simulink model "ackerman_ROS_neural_controller_v2"  (R2023a)
settings: Solver=FixedStepDiscrete  StartTime=0.0  StopTime=200  FixedStep=0.1  RelTol=1e-3
undefined symbols (not defined in the file or in its folder): Angular, Linear
libraries: neural x413, robotlib x15, robotcorelib x1
(part 8 of 17)

== system ackerman_ROS_neural_controller_v2/ME ENCANTA/Layer 1/IW{1,1} ==
  "pd{1,1}" : Inport  PortDimensions=8  SampleTime=0.1
      mask Display: e = 0.06;c1 = [120 230 180]/255;c2 = ([120 230 180]+0)/(256+128);c3 = ([120 230 180]+128)/(256+128);patch([0 1 1 0],[0 0 1 1],c1);patch([0 1 1 1-e 1-e 0+e],[0 0 1 1-e 0+e 0+e],c2);patch([0 0 1 1-e 0+e 0+e],[0 1 1 1-e 1-e 0+e],c3);plot([0 1 1 0 0],[0 0 1 1 0]);
  "IW{1,1}(1,:)'" : Constant  Value=[0.971980235182158924800432941992767155170440673828125;2.567078221588861453028584946878254413604736328125;-0.0638964923073234991601765386803890578448772430419921875;0.187982900118411178080890522323898039758205413818359375;1.435142271716796091851620076340623199939727783203125;-1.2440064926958480651109084647032432258129119873046875;-1.715625221300081104658374897553585469722747802734375;-0.3178705401241617156671281918534077703952789306640625]
      mask Display: e = 0.06;c1 = [120 150 230]/255;c2 = ([120 150 230]+0)/383;c3 = ([120 150 230]+128)/383;patch([0 1 1 0],[0 0 1 1],c1);patch([0 1 1 1-e 1-e 0+e],[0 0 1 1-e 0+e 0+e],c2);patch([0 0 1 1-e 0+e 0+e],[0 1 1 1-e 1-e 0+e],c3);plot([0 1 1 0 0],[0 0 1 1 0]);disp('Weights');
  "IW{1,1}(10,:)'" : Constant  Value=[0.952957574863269929466014218633063137531280517578125;-1.279752017667800334521643890184350311756134033203125;-0.780817996752551923833607361302711069583892822265625;-0.73631471257776326400090738388826139271259307861328125;0.279679452980061415967583116071182303130626678466796875;1.76479096051938189049224092741496860980987548828125;-0.41872113667667931746763088085572235286235809326171875;-0.269270961130175290332289250727626495063304901123046875]
      mask Display: e = 0.06;c1 = [120 150 230]/255;c2 = ([120 150 230]+0)/383;c3 = ([120 150 230]+128)/383;patch([0 1 1 0],[0 0 1 1],c1);patch([0 1 1 1-e 1-e 0+e],[0 0 1 1-e 0+e 0+e],c2);patch([0 0 1 1-e 0+e 0+e],[0 1 1 1-e 1-e 0+e],c3);plot([0 1 1 0 0],[0 0 1 1 0]);disp('Weights');
  "IW{1,1}(11,:)'" : Constant  Value=[-0.7943142555522564318692957385792396962642669677734375;-0.54810133824739093455491456552408635616302490234375;-0.0209028643619187902424894076602868153713643550872802734375;0.207116084413179468715071607221034355461597442626953125;1.4609012214747443270113080870942212641239166259765625;-0.94419545667940074640256398197379894554615020751953125;-1.49407969221122893799247322021983563899993896484375;0.36046049644091560093528414654429070651531219482421875]
      mask Display: e = 0.06;c1 = [120 150 230]/255;c2 = ([120 150 230]+0)/383;c3 = ([120 150 230]+128)/383;patch([0 1 1 0],[0 0 1 1],c1);patch([0 1 1 1-e 1-e 0+e],[0 0 1 1-e 0+e 0+e],c2);patch([0 0 1 1-e 0+e 0+e],[0 1 1 1-e 1-e 0+e],c3);plot([0 1 1 0 0],[0 0 1 1 0]);disp('Weights');
  "IW{1,1}(12,:)'" : Constant  Value=[-1.63964337746614763346997278858907520771026611328125;0.60076169030219350730703808949328958988189697265625;0.71625941833236861366884795643272809684276580810546875;0.28432619515038293211972586504998616874217987060546875;1.008858171661137337338232100591994822025299072265625;1.226017776539758852294426105800084769725799560546875;-1.7365630219620447061146251144236885011196136474609375;-0.429447135602839313861522896331734955310821533203125]
      mask Display: e = 0.06;c1 = [120 150 230]/255;c2 = ([120 150 230]+0)/383;c3 = ([120 150 230]+128)/383;patch([0 1 1 0],[0 0 1 1],c1);patch([0 1 1 1-e 1-e 0+e],[0 0 1 1-e 0+e 0+e],c2);patch([0 0 1 1-e 0+e 0+e],[0 1 1 1-e 1-e 0+e],c3);plot([0 1 1 0 0],[0 0 1 1 0]);disp('Weights');
  "IW{1,1}(13,:)'" : Constant  Value=[-0.046458660075713177628475847313893609680235385894775390625;1.309328092935980958344543978455476462841033935546875;-0.2053412555322882138142404073732905089855194091796875;-1.0241502298471925058720444212667644023895263671875;0.33819473753734718979302442676271311938762664794921875;1.500511362857012809257639673887751996517181396484375;0.89838152047738495387108059730962850153446197509765625;0.38963898857398138186880487410235218703746795654296875]
      mask Display: e = 0.06;c1 = [120 150 230]/255;c2 = ([120 150 230]+0)/383;c3 = ([120 150 230]+128)/383;patch([0 1 1 0],[0 0 1 1],c1);patch([0 1 1 1-e 1-e 0+e],[0 0 1 1-e 0+e 0+e],c2);patch([0 0 1 1-e 0+e 0+e],[0 1 1 1-e 1-e 0+e],c3);plot([0 1 1 0 0],[0 0 1 1 0]);disp('Weights');
  "IW{1,1}(14,:)'" : Constant  Value=[-0.835126481572200152214691115659661591053009033203125;0.67771081724395265677429733841563574969768524169921875;0.32746319190107009422519013241981156170368194580078125;0.496135681159649621907448135971208103001117706298828125;-0.77500849546231187492395520166610367596149444580078125;-0.53766641721378238827355744433589279651641845703125;0.354972473239116237397894337846082635223865509033203125;1.312743418109337145693871207186020910739898681640625]
      mask Display: e = 0.06;c1 = [120 150 230]/255;c2 = ([120 150 230]+0)/383;c3 = ([120 150 230]+128)/383;patch([0 1 1 0],[0 0 1 1],c1);patch([0 1 1 1-e 1-e 0+e],[0 0 1 1-e 0+e 0+e],c2);patch([0 0 1 1-e 0+e 0+e],[0 1 1 1-e 1-e 0+e],c3);plot([0 1 1 0 0],[0 0 1 1 0]);disp('Weights');
  "IW{1,1}(15,:)'" : Constant  Value=[-0.18608216993497517233180360562982968986034393310546875;-0.67339069859827649366934565478004515171051025390625;0.286183692221986085701956881166552193462848663330078125;0.90019583556312310346214644596329890191555023193359375;-1.424886791004641661828600263106636703014373779296875;-0.552278192782113652725684005417861044406890869140625;-0.58322513421994226501254843242350034415721893310546875;0.71811307953740766141237372721661813557147979736328125]
      mask Display: e = 0.06;c1 = [120 150 230]/255;c2 = ([120 150 230]+0)/383;c3 = ([120 150 230]+128)/383;patch([0 1 1 0],[0 0 1 1],c1);patch([0 1 1 1-e 1-e 0+e],[0 0 1 1-e 0+e 0+e],c2);patch([0 0 1 1-e 0+e 0+e],[0 1 1 1-e 1-e 0+e],c3);plot([0 1 1 0 0],[0 0 1 1 0]);disp('Weights');
  "IW{1,1}(2,:)'" : Constant  Value=[-1.35611856667662333819635023246519267559051513671875;-0.6596259355066333984751736352336592972278594970703125;-2.15308333009377150801810785196721553802490234375;-0.594254710313253386999576832749880850315093994140625;1.183809903206018088184237058158032596111297607421875;1.3778074261582233805967234729905612766742706298828125;-0.4951736029469759881038726234692148864269256591796875;-0.5083250892003707832600412075407803058624267578125]
      mask Display: e = 0.06;c1 = [120 150 230]/255;c2 = ([120 150 230]+0)/383;c3 = ([120 150 230]+128)/383;patch([0 1 1 0],[0 0 1 1],c1);patch([0 1 1 1-e 1-e 0+e],[0 0 1 1-e 0+e 0+e],c2);patch([0 0 1 1-e 0+e 0+e],[0 1 1 1-e 1-e 0+e],c3);plot([0 1 1 0 0],[0 0 1 1 0]);disp('Weights');
  "IW{1,1}(3,:)'" : Constant  Value=[0.389330121892868863398007306386716663837432861328125;0.2289315734305190641606486678938381373882293701171875;0.68045717842820419019034261509659700095653533935546875;-0.72428464448281071330626446069800294935703277587890625;-3.111683839695417841397784286527894437313079833984375;1.8061369740664001692920237474027089774608612060546875;2.901306769919713257621651791851036250591278076171875;-0.165240155407275712828862879177904687821865081787109375]
      mask Display: e = 0.06;c1 = [120 150 230]/255;c2 = ([120 150 230]+0)/383;c3 = ([120 150 230]+128)/383;patch([0 1 1 0],[0 0 1 1],c1);patch([0 1 1 1-e 1-e 0+e],[0 0 1 1-e 0+e 0+e],c2);patch([0 0 1 1-e 0+e 0+e],[0 1 1 1-e 1-e 0+e],c3);plot([0 1 1 0 0],[0 0 1 1 0]);disp('Weights');
  "IW{1,1}(4,:)'" : Constant  Value=[1.6848774452106629606618071193224750459194183349609375;-0.2113971201403252175854419192546629346907138824462890625;-0.40644343158014095696017875525285489857196807861328125;0.98312175830758985473067923521739430725574493408203125;1.5222720525634070298792721587233245372772216796875;0.37693409531385524413593657300225459039211273193359375;0.2450165084343079169304502329396200366318225860595703125;-0.760503980708643556596371126943267881870269775390625]
      mask Display: e = 0.06;c1 = [120 150 230]/255;c2 = ([120 150 230]+0)/383;c3 = ([120 150 230]+128)/383;patch([0 1 1 0],[0 0 1 1],c1);patch([0 1 1 1-e 1-e 0+e],[0 0 1 1-e 0+e 0+e],c2);patch([0 0 1 1-e 0+e 0+e],[0 1 1 1-e 1-e 0+e],c3);plot([0 1 1 0 0],[0 0 1 1 0]);disp('Weights');
  "IW{1,1}(5,:)'" : Constant  Value=[1.7316373522789654249010027342592366039752960205078125;1.2495315454890889572681089703110046684741973876953125;1.1345171396436393163043021559133194386959075927734375;0.55816746854987309145457174963667057454586029052734375;0.336413043621611784761427088596974499523639678955078125;-0.6475244665177035674474836923764087259769439697265625;1.2412636084071022590791244510910473763942718505859375;-0.45205615342753124874519699005759321153163909912109375]
      mask Display: e = 0.06;c1 = [120 150 230]/255;c2 = ([120 150 230]+0)/383;c3 = ([120 150 230]+128)/383;patch([0 1 1 0],[0 0 1 1],c1);patch([0 1 1 1-e 1-e 0+e],[0 0 1 1-e 0+e 0+e],c2);patch([0 0 1 1-e 0+e 0+e],[0 1 1 1-e 1-e 0+e],c3);plot([0 1 1 0 0],[0 0 1 1 0]);disp('Weights');
  "IW{1,1}(6,:)'" : Constant  Value=[-0.1509239964485774854185962112751440145075321197509765625;-1.19586695150943089771544691757299005985260009765625;0.80360230515575514775861165617243386805057525634765625;-0.6183180438151278934810761711560189723968505859375;1.2181859235617549241936785620055161416530609130859375;-1.402058986093745573953128769062459468841552734375;2.21178431671591813056920727831311523914337158203125;5.8493224896000324264377923100255429744720458984375]
      mask Display: e = 0.06;c1 = [120 150 230]/255;c2 = ([120 150 230]+0)/383;c3 = ([120 150 230]+128)/383;patch([0 1 1 0],[0 0 1 1],c1);patch([0 1 1 1-e 1-e 0+e],[0 0 1 1-e 0+e 0+e],c2);patch([0 0 1 1-e 0+e 0+e],[0 1 1 1-e 1-e 0+e],c3);plot([0 1 1 0 0],[0 0 1 1 0]);disp('Weights');
  "IW{1,1}(7,:)'" : Constant  Value=[0.8609195814912504740590293295099399983882904052734375;-2.130317054986762048685022818972356617450714111328125;-0.056947587820770355360178172077212366275489330291748046875;0.327433012969035319716937237899401225149631500244140625;0.2186081327389498285551638900869875214993953704833984375;-1.036658261972080996571321520605124533176422119140625;2.47996978858621286434527064557187259197235107421875;-1.953257557304577840540105171385221183300018310546875]
      mask Display: e = 0.06;c1 = [120 150 230]/255;c2 = ([120 150 230]+0)/383;c3 = ([120 150 230]+128)/383;patch([0 1 1 0],[0 0 1 1],c1);patch([0 1 1 1-e 1-e 0+e],[0 0 1 1-e 0+e 0+e],c2);patch([0 0 1 1-e 0+e 0+e],[0 1 1 1-e 1-e 0+e],c3);plot([0 1 1 0 0],[0 0 1 1 0]);disp('Weights');
  "IW{1,1}(8,:)'" : Constant  Value=[-0.46388264526166789192274109154823236167430877685546875;-0.5661191272907097893352101891650818288326263427734375;-0.181870215050510652954329771091579459607601165771484375;0.300246660440473822628604239071137271821498870849609375;-0.025378748936564408944516202382146730087697505950927734375;1.61731333714226455100515522644855082035064697265625;1.5124425407989434688715846277773380279541015625;-0.1772881404680668737672277757155825383961200714111328125]
      mask Display: e = 0.06;c1 = [120 150 230]/255;c2 = ([120 150 230]+0)/383;c3 = ([120 150 230]+128)/383;patch([0 1 1 0],[0 0 1 1],c1);patch([0 1 1 1-e 1-e 0+e],[0 0 1 1-e 0+e 0+e],c2);patch([0 0 1 1-e 0+e 0+e],[0 1 1 1-e 1-e 0+e],c3);plot([0 1 1 0 0],[0 0 1 1 0]);disp('Weights');
  "IW{1,1}(9,:)'" : Constant  Value=[-0.061268372693201796075346265979533200152218341827392578125;-0.419245737318853561870213297879672609269618988037109375;1.2976808489538809165964039493701420724391937255859375;-0.36556525140667073259237440652213990688323974609375;-1.8561266888005982789167092050774954259395599365234375;-0.7655307190718494414483075161115266382694244384765625;0.70605083757586839521280808185110799968242645263671875;-1.19981392938518727220298387692309916019439697265625]
      mask Display: e = 0.06;c1 = [120 150 230]/255;c2 = ([120 150 230]+0)/383;c3 = ([120 150 230]+128)/383;patch([0 1 1 0],[0 0 1 1],c1);patch([0 1 1 1-e 1-e 0+e],[0 0 1 1-e 0+e 0+e],c2);patch([0 0 1 1-e 0+e 0+e],[0 1 1 1-e 1-e 0+e],c3);plot([0 1 1 0 0],[0 0 1 1 0]);disp('Weights');
  Mux : Mux  Inputs=15
      mask Display: e = 0.06;c1 = [120 150 230]/255;c2 = ([120 150 230]+0)/383;c3 = ([120 150 230]+128)/383;patch([0 1 1 0],[0 0 1 1],c1);patch([0 1 1 1-e 1-e 0+e],[0 0 1 1-e 0+e 0+e],c2);patch([0 0 1 1-e 0+e 0+e],[0 1 1 1-e 1-e 0+e],c3);plot([0 1 1 0 0],[0 0 1 1 0]);disp('Mux');
  dotprod{1..15} (15 alike) : neural/Weight Functions/dotprod
  "iz{1,1}" : Outport
      mask Display: e = 0.06;c1 = [120 230 180]/255;c2 = ([120 230 180]+0)/(256+128);c3 = ([120 230 180]+128)/(256+128);patch([0 1 1 0],[0 0 1 1],c1);patch([0 1 1 1-e 1-e 0+e],[0 0 1 1-e 0+e 0+e],c2);patch([0 0 1 1-e 0+e 0+e],[0 1 1 1-e 1-e 0+e],c3);plot([0 1 1 0 0],[0 0 1 1 0]);
  wires:
  "IW{1,1}(1,:)'"/1 -> dotprod1/1
  "pd{1,1}"/1 -> dotprod1/2, dotprod2/2, dotprod3/2, dotprod4/2, dotprod5/2, dotprod6/2, dotprod7/2, dotprod8/2, dotprod9/2, dotprod10/2, dotprod11/2, dotprod12/2, dotprod13/2, dotprod14/2, dotprod15/2
  dotprod1/1 -> Mux/1
  "IW{1,1}(2,:)'"/1 -> dotprod2/1
  dotprod2/1 -> Mux/2
  "IW{1,1}(3,:)'"/1 -> dotprod3/1
  dotprod3/1 -> Mux/3
  "IW{1,1}(4,:)'"/1 -> dotprod4/1
  dotprod4/1 -> Mux/4
  "IW{1,1}(5,:)'"/1 -> dotprod5/1
  dotprod5/1 -> Mux/5
  "IW{1,1}(6,:)'"/1 -> dotprod6/1
  dotprod6/1 -> Mux/6
  "IW{1,1}(7,:)'"/1 -> dotprod7/1
  dotprod7/1 -> Mux/7
  "IW{1,1}(8,:)'"/1 -> dotprod8/1
  dotprod8/1 -> Mux/8
  "IW{1,1}(9,:)'"/1 -> dotprod9/1
  dotprod9/1 -> Mux/9
  "IW{1,1}(10,:)'"/1 -> dotprod10/1
  dotprod10/1 -> Mux/10
  "IW{1,1}(11,:)'"/1 -> dotprod11/1
  dotprod11/1 -> Mux/11
  "IW{1,1}(12,:)'"/1 -> dotprod12/1
  dotprod12/1 -> Mux/12
  "IW{1,1}(13,:)'"/1 -> dotprod13/1
  dotprod13/1 -> Mux/13
  "IW{1,1}(14,:)'"/1 -> dotprod14/1
  dotprod14/1 -> Mux/14
  "IW{1,1}(15,:)'"/1 -> dotprod15/1
  dotprod15/1 -> Mux/15
  Mux/1 -> "iz{1,1}"/1

== system ackerman_ROS_neural_controller_v2/ME ENCANTA/Layer 2/Delays 1 ==
  "p{2}" : Inport  PortDimensions=15  SampleTime=0.1
      mask Display: e = 0.06;c1 = [120 230 180]/255;c2 = ([120 230 180]+0)/(256+128);c3 = ([120 230 180]+128)/(256+128);patch([0 1 1 0],[0 0 1 1],c1);patch([0 1 1 1-e 1-e 0+e],[0 0 1 1-e 0+e 0+e],c2);patch([0 0 1 1-e 0+e 0+e],[0 1 1 1-e 1-e 0+e],c3);plot([0 1 1 0 0],[0 0 1 1 0]);
  mux : Mux  Inputs=1
      mask Display: e = 0.06;c1 = [120 150 230]/255;c2 = ([120 150 230]+0)/383;c3 = ([120 150 230]+128)/383;patch([0 1 1 0],[0 0 1 1],c1);patch([0 1 1 1-e 1-e 0+e],[0 0 1 1-e 0+e 0+e],c2);patch([0 0 1 1-e 0+e 0+e],[0 1 1 1-e 1-e 0+e],c3);plot([0 1 1 0 0],[0 0 1 1 0]);disp('Mux')
  "pd{2,1}" : Outport
      mask Display: e = 0.06;c1 = [120 230 180]/255;c2 = ([120 230 180]+0)/(256+128);c3 = ([120 230 180]+128)/(256+128);patch([0 1 1 0],[0 0 1 1],c1);patch([0 1 1 1-e 1-e 0+e],[0 0 1 1-e 0+e 0+e],c2);patch([0 0 1 1-e 0+e 0+e],[0 1 1 1-e 1-e 0+e],c3);plot([0 1 1 0 0],[0 0 1 1 0]);
  wires:
  "p{2}"/1 -> mux/1
  mux/1 -> "pd{2,1}"/1

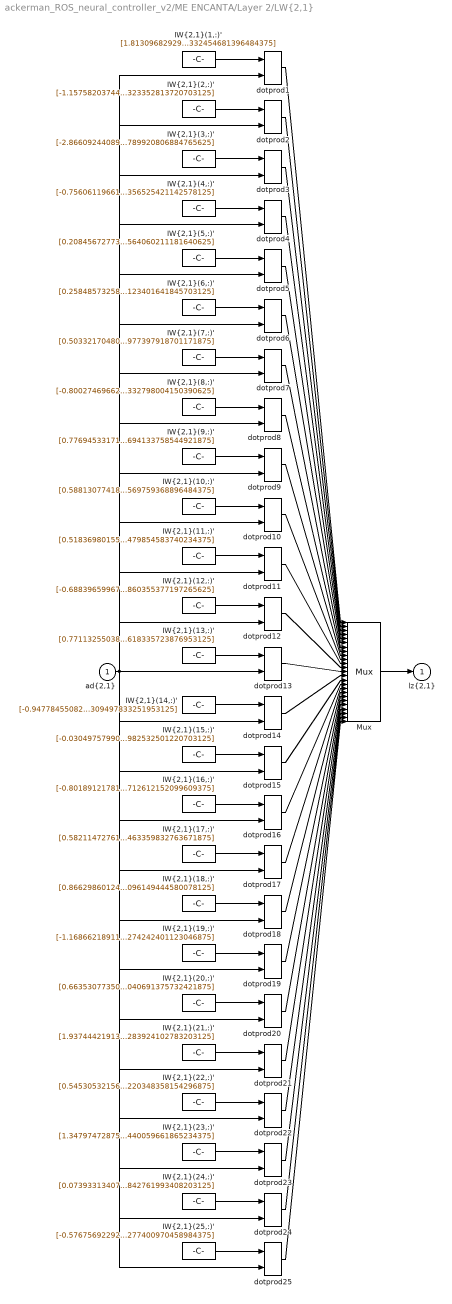
== system ackerman_ROS_neural_controller_v2/ME ENCANTA/Layer 2/LW{2,1} ==
  "ad{2,1}" : Inport  PortDimensions=15  SampleTime=0.1
      mask Display: e = 0.06;c1 = [120 230 180]/255;c2 = ([120 230 180]+0)/(256+128);c3 = ([120 230 180]+128)/(256+128);patch([0 1 1 0],[0 0 1 1],c1);patch([0 1 1 1-e 1-e 0+e],[0 0 1 1-e 0+e 0+e],c2);patch([0 0 1 1-e 0+e 0+e],[0 1 1 1-e 1-e 0+e],c3);plot([0 1 1 0 0],[0 0 1 1 0]);
  "IW{2,1}(1,:)'" : Constant  Value=[1.8130968292963027810316134491586126387119293212890625;-0.255772831790393395667848608354688622057437896728515625;1.8095842791136875771229597376077435910701751708984375;0.7936575422578329153111553750932216644287109375;0.092670501554258988274881403413019143044948577880859375;0.6296319508271845943880862250807695090770721435546875;0.541757471966922476980244027799926698207855224609375;0.44501774222277779013978715738630853593349456787109375;-0.71599648125620418692705015928368084132671356201171875;-0.371588811241314431743631985227693803608417510986328125;1.247768693986584853661270244629122316837310791015625;0.53497004586812824111774489210802130401134490966796875;1.1381736231371848422355697039165534079074859619140625;-0.7106397226316072401886003717663697898387908935546875;-0.27517285573338357007600052384077571332454681396484375]
      mask Display: e = 0.06;c1 = [120 150 230]/255;c2 = ([120 150 230]+0)/383;c3 = ([120 150 230]+128)/383;patch([0 1 1 0],[0 0 1 1],c1);patch([0 1 1 1-e 1-e 0+e],[0 0 1 1-e 0+e 0+e],c2);patch([0 0 1 1-e 0+e 0+e],[0 1 1 1-e 1-e 0+e],c3);plot([0 1 1 0 0],[0 0 1 1 0]);disp('weights');
  "IW{2,1}(10,:)'" : Constant  Value=[0.588130774187691773846609066822566092014312744140625;-0.339759906672265798999177377481828443706035614013671875;-0.0228880925425688323826545200745385955087840557098388671875;1.4178785693877216100844407264958135783672332763671875;-0.6795640976779804276475260849110782146453857421875;0.0765118726073720500924224552363739348948001861572265625;-0.8237439875990937299121696923975832760334014892578125;-0.8653789643172740131404907515388913452625274658203125;1.2355083598950520329395885710255242884159088134765625;0.11697653409674797775341659189507481642067432403564453125;1.0095133312632242894579803760279901325702667236328125;0.353335780949750877244497360152308829128742218017578125;-0.81331883035691188155169584206305444240570068359375;-0.3449343897329091301884318454540334641933441162109375;0.0585989005349679403789053822038113139569759368896484375]
      mask Display: e = 0.06;c1 = [120 150 230]/255;c2 = ([120 150 230]+0)/383;c3 = ([120 150 230]+128)/383;patch([0 1 1 0],[0 0 1 1],c1);patch([0 1 1 1-e 1-e 0+e],[0 0 1 1-e 0+e 0+e],c2);patch([0 0 1 1-e 0+e 0+e],[0 1 1 1-e 1-e 0+e],c3);plot([0 1 1 0 0],[0 0 1 1 0]);disp('weights');
  "IW{2,1}(11,:)'" : Constant  Value=[0.51836980155931133840141455948469229042530059814453125;-0.2263315686119481140448073119841865263879299163818359375;0.25026052405077781060072084073908627033233642578125;-1.1991198499209947403443266011890955269336700439453125;0.19636284461798769740425996133126318454742431640625;-0.6854097603523439108386128282290883362293243408203125;-0.34742080057330448905617004129453562200069427490234375;0.44970384640605953752157120106858201324939727783203125;-1.2052694498838347758606914794654585421085357666015625;-0.394952424568869420173911066740402020514011383056640625;0.416458575533069363938665219393442384898662567138671875;0.6064257071360328321674160179099999368190765380859375;-0.53127670999813603192052369195153005421161651611328125;-0.56277449650893063282097728006192483007907867431640625;-0.153180536621822349641064420211478136479854583740234375]
      mask Display: e = 0.06;c1 = [120 150 230]/255;c2 = ([120 150 230]+0)/383;c3 = ([120 150 230]+128)/383;patch([0 1 1 0],[0 0 1 1],c1);patch([0 1 1 1-e 1-e 0+e],[0 0 1 1-e 0+e 0+e],c2);patch([0 0 1 1-e 0+e 0+e],[0 1 1 1-e 1-e 0+e],c3);plot([0 1 1 0 0],[0 0 1 1 0]);disp('weights');
  "IW{2,1}(12,:)'" : Constant  Value=[-0.6883965996711751689218772298772819340229034423828125;0.35374993021716349961280911884387023746967315673828125;-0.64690670192794119675028241545078344643115997314453125;-1.244175327075421666478405313682742416858673095703125;-1.027393066228861062683108684723265469074249267578125;0.0980377263800632781087784906048909761011600494384765625;-1.6922461507361108434821517221280373632907867431640625;-0.8175833332197550706865740721696056425571441650390625;0.46281195349833870178457573274499736726284027099609375;0.65038188859338619263184000374167226254940032958984375;0.1770483528829895902845237287692725658416748046875;0.4494192019014533467924366050283424556255340576171875;0.5996086064405259374865408972254954278469085693359375;-0.67548041085466337118958790597389452159404754638671875;-0.2116819913559425947457981465049670077860355377197265625]
      mask Display: e = 0.06;c1 = [120 150 230]/255;c2 = ([120 150 230]+0)/383;c3 = ([120 150 230]+128)/383;patch([0 1 1 0],[0 0 1 1],c1);patch([0 1 1 1-e 1-e 0+e],[0 0 1 1-e 0+e 0+e],c2);patch([0 0 1 1-e 0+e 0+e],[0 1 1 1-e 1-e 0+e],c3);plot([0 1 1 0 0],[0 0 1 1 0]);disp('weights');
  "IW{2,1}(13,:)'" : Constant  Value=[0.77113255038470962521301999004208482801914215087890625;0.75428016356330307434774340435978956520557403564453125;0.75009868465519147218145690203527919948101043701171875;-0.09961538321190703537677535450711729936301708221435546875;0.11868437831724436282154755417650449089705944061279296875;0.52094326685391434406113830846152268350124359130859375;0.442267979911934394632311295936233364045619964599609375;0.845822317486990105095401304424740374088287353515625;-0.2674678094433160513432312654913403093814849853515625;0.10215715573276136496350119386988808400928974151611328125;0.64768638710050840945342542909202165901660919189453125;-0.557712680196601695570279844105243682861328125;1.1950428157187402700145639755646698176860809326171875;0.0790607204794342710574284183167037554085254669189453125;0.160681987458118957778907542888191528618335723876953125]
      mask Display: e = 0.06;c1 = [120 150 230]/255;c2 = ([120 150 230]+0)/383;c3 = ([120 150 230]+128)/383;patch([0 1 1 0],[0 0 1 1],c1);patch([0 1 1 1-e 1-e 0+e],[0 0 1 1-e 0+e 0+e],c2);patch([0 0 1 1-e 0+e 0+e],[0 1 1 1-e 1-e 0+e],c3);plot([0 1 1 0 0],[0 0 1 1 0]);disp('weights');
  "IW{2,1}(14,:)'" : Constant  Value=[-0.9477845508233488924787479845690540969371795654296875;-0.040494110400246120795575421880130306817591190338134765625;0.2287797520309740040289625540026463568210601806640625;0.6167074035373534268700268512475304305553436279296875;-0.2350520581197346192681152388104237616062164306640625;-1.3281227076352111193813243517070077359676361083984375;-0.1178795834398659037045575814772746525704860687255859375;-0.74520043189864926258536570458090864121913909912109375;-0.6159653204494162093141085279057733714580535888671875;0.7566462781938838588757789693772792816162109375;-0.3343066054293888367254794502514414489269256591796875;-0.255998734879846867595887260904419235885143280029296875;0.033943809716176935598053177045585471205413341522216796875;0.048952723824412978925746386948958388529717922210693359375;0.67881404179711613000591796662774868309497833251953125]
      mask Display: e = 0.06;c1 = [120 150 230]/255;c2 = ([120 150 230]+0)/383;c3 = ([120 150 230]+128)/383;patch([0 1 1 0],[0 0 1 1],c1);patch([0 1 1 1-e 1-e 0+e],[0 0 1 1-e 0+e 0+e],c2);patch([0 0 1 1-e 0+e 0+e],[0 1 1 1-e 1-e 0+e],c3);plot([0 1 1 0 0],[0 0 1 1 0]);disp('weights');
  "IW{2,1}(15,:)'" : Constant  Value=[-0.03049757990487182712779912208134192042052745819091796875;0.9800327508020298949986681691370904445648193359375;-1.8904627904007345051695665461011230945587158203125;1.692716332211109619976241447147913277149200439453125;-0.4149057584485833505283380873152054846286773681640625;-1.6408767559287034121240367312566377222537994384765625;0.0951327642375493776061290418510907329618930816650390625;0.589782682203221053640618265490047633647918701171875;0.85295844649167251727561733787297271192073822021484375;-0.033560316239322325604366170637149480171501636505126953125;-0.1290250183905295722208705910816206596791744232177734375;-1.1713690917720551709635401493869721889495849609375;-0.410450607875675499425227599203935824334621429443359375;-0.86691201708639076262130629402236081659793853759765625;0.57207519575668552835878699625027365982532501220703125]
      mask Display: e = 0.06;c1 = [120 150 230]/255;c2 = ([120 150 230]+0)/383;c3 = ([120 150 230]+128)/383;patch([0 1 1 0],[0 0 1 1],c1);patch([0 1 1 1-e 1-e 0+e],[0 0 1 1-e 0+e 0+e],c2);patch([0 0 1 1-e 0+e 0+e],[0 1 1 1-e 1-e 0+e],c3);plot([0 1 1 0 0],[0 0 1 1 0]);disp('weights');
  "IW{2,1}(16,:)'" : Constant  Value=[-0.80189121781496519592025151723646558821201324462890625;-0.78812392539758524545590034904307685792446136474609375;0.1840930035032713740772436494808061979711055755615234375;-0.038169568744800229376235023437402560375630855560302734375;-0.159736986304258532509692258827271871268749237060546875;0.2474929546816186931579295560368336737155914306640625;-0.339351274836662053502323033171705901622772216796875;-0.70085419640267598850869035231880843639373779296875;-0.328571349899448417186675897028180770576000213623046875;0.05047858631007358376496796381616150029003620147705078125;0.6475496758696106525121649610809981822967529296875;0.1817661991711687630157712192158214747905731201171875;0.50521990515887493788937945282668806612491607666015625;1.24856011086177165481103656929917633533477783203125;0.38109976536721779094563089529401622712612152099609375]
      mask Display: e = 0.06;c1 = [120 150 230]/255;c2 = ([120 150 230]+0)/383;c3 = ([120 150 230]+128)/383;patch([0 1 1 0],[0 0 1 1],c1);patch([0 1 1 1-e 1-e 0+e],[0 0 1 1-e 0+e 0+e],c2);patch([0 0 1 1-e 0+e 0+e],[0 1 1 1-e 1-e 0+e],c3);plot([0 1 1 0 0],[0 0 1 1 0]);disp('weights');
  "IW{2,1}(17,:)'" : Constant  Value=[0.582114727618114446983099696808494627475738525390625;0.4113077821994697291785314519074745476245880126953125;0.475252633760660014861088029647362418472766876220703125;-0.243515994374020106061351498283329419791698455810546875;0.1813843290805878527560679458474623970687389373779296875;0.032086722982967053052760775244678370654582977294921875;0.242124293417356195590173228993080556392669677734375;0.5660862521343184017297289756243117153644561767578125;0.298156848781912398038684841594658792018890380859375;-1.5344952127159354748897612807922996580600738525390625;0.53500301355363200084269692524685524404048919677734375;-0.1748285988811624502847763551471871323883533477783203125;-0.55881399566798373168552416245802305638790130615234375;-0.67109134490484090296291697086417116224765777587890625;-0.74402615771247837539448255483875982463359832763671875]
      mask Display: e = 0.06;c1 = [120 150 230]/255;c2 = ([120 150 230]+0)/383;c3 = ([120 150 230]+128)/383;patch([0 1 1 0],[0 0 1 1],c1);patch([0 1 1 1-e 1-e 0+e],[0 0 1 1-e 0+e 0+e],c2);patch([0 0 1 1-e 0+e 0+e],[0 1 1 1-e 1-e 0+e],c3);plot([0 1 1 0 0],[0 0 1 1 0]);disp('weights');
  "IW{2,1}(18,:)'" : Constant  Value=[0.86629860124357538353478958015330135822296142578125;0.468578113618298541798168344030273146927356719970703125;-0.191154806197775750664646920995437540113925933837890625;-0.310719341612152033516025539938709698617458343505859375;-0.46879073947875771199989003434893675148487091064453125;0.66883578383566366643009359904681332409381866455078125;-0.41297906470973799741841503418982028961181640625;0.344036592633888582692947011310025118291378021240234375;-0.42057896979676023807570572898839600384235382080078125;-0.283333125147997966220003718262887559831142425537109375;-0.7723200332906248188891140671330504119396209716796875;-0.47611908559641780147586587190744467079639434814453125;0.76423719315329263768177270321757532656192779541015625;0.1342166940656241147511451572427176870405673980712890625;0.381964959240758183955932736353133805096149444580078125]
      mask Display: e = 0.06;c1 = [120 150 230]/255;c2 = ([120 150 230]+0)/383;c3 = ([120 150 230]+128)/383;patch([0 1 1 0],[0 0 1 1],c1);patch([0 1 1 1-e 1-e 0+e],[0 0 1 1-e 0+e 0+e],c2);patch([0 0 1 1-e 0+e 0+e],[0 1 1 1-e 1-e 0+e],c3);plot([0 1 1 0 0],[0 0 1 1 0]);disp('weights');
  "IW{2,1}(19,:)'" : Constant  Value=[-1.168662189116980609782103783800266683101654052734375;0.118042226085451285033656176892691291868686676025390625;-0.2802798218159716636677103451802395284175872802734375;1.047610055646647442273433625814504921436309814453125;0.214264467796893398610080794242094270884990692138671875;0.13401333461403208691109512074035592377185821533203125;0.1483592389191067673070989485495374538004398345947265625;0.21371412461797245629924191234749741852283477783203125;-0.153162771539127773312571889618993736803531646728515625;0.349827990979937830662294118155841715633869171142578125;0.8211905905739715905156117514707148075103759765625;0.398052304941000023585928602187777869403362274169921875;-0.23662395538542690953676128629012964665889739990234375;-0.439546017544050815484268923682975582778453826904296875;0.6530566614403194858340384598704986274242401123046875]
      mask Display: e = 0.06;c1 = [120 150 230]/255;c2 = ([120 150 230]+0)/383;c3 = ([120 150 230]+128)/383;patch([0 1 1 0],[0 0 1 1],c1);patch([0 1 1 1-e 1-e 0+e],[0 0 1 1-e 0+e 0+e],c2);patch([0 0 1 1-e 0+e 0+e],[0 1 1 1-e 1-e 0+e],c3);plot([0 1 1 0 0],[0 0 1 1 0]);disp('weights');
  "IW{2,1}(2,:)'" : Constant  Value=[-1.1575820374496199605118817999027669429779052734375;-0.6276412292356301492191050783731043338775634765625;1.8191819355073517439080887925229035317897796630859375;-0.17860930203348124312157096937880851328372955322265625;0.89845398519739294584951494471170008182525634765625;-0.1157393396725430456672967238773708231747150421142578125;0.7761914429547240867890423032804392278194427490234375;-0.011287593590528166576092417017207480967044830322265625;0.268655522803954049937402714931522496044635772705078125;0.182392483408585104331933735011261887848377227783203125;0.63888010521827409693429444814682938158512115478515625;-0.050615611392042701710547447646604268811643123626708984375;-0.393408062322786966635845828932360745966434478759765625;0.07753455937068576275805753539316356182098388671875;-0.48516144923123949439514035475440323352813720703125]
      mask Display: e = 0.06;c1 = [120 150 230]/255;c2 = ([120 150 230]+0)/383;c3 = ([120 150 230]+128)/383;patch([0 1 1 0],[0 0 1 1],c1);patch([0 1 1 1-e 1-e 0+e],[0 0 1 1-e 0+e 0+e],c2);patch([0 0 1 1-e 0+e 0+e],[0 1 1 1-e 1-e 0+e],c3);plot([0 1 1 0 0],[0 0 1 1 0]);disp('weights');
  "IW{2,1}(20,:)'" : Constant  Value=[0.663530773507981397330013351165689527988433837890625;0.357190282104396350515429503502673469483852386474609375;-0.59535926114223247651580095407553017139434814453125;-0.9324157483475052909938085576868616044521331787109375;0.60718787255547324033244649399421177804470062255859375;-0.6979877164513508258636420578113757073879241943359375;-0.43086321636308955174143875410663895308971405029296875;0.280996744886260974016778391160187311470508575439453125;0.1620797880726918827054561234035645611584186553955078125;-0.3221208785097082749615537977661006152629852294921875;0.307649344062845220282298441816237755119800567626953125;0.3456444268407352637950680218636989593505859375;0.102343039410194347471616538314265199005603790283203125;-0.463147189297440642352654549540602602064609527587890625;-0.7625829682402744946756456556613557040691375732421875]
      mask Display: e = 0.06;c1 = [120 150 230]/255;c2 = ([120 150 230]+0)/383;c3 = ([120 150 230]+128)/383;patch([0 1 1 0],[0 0 1 1],c1);patch([0 1 1 1-e 1-e 0+e],[0 0 1 1-e 0+e 0+e],c2);patch([0 0 1 1-e 0+e 0+e],[0 1 1 1-e 1-e 0+e],c3);plot([0 1 1 0 0],[0 0 1 1 0]);disp('weights');
  "IW{2,1}(21,:)'" : Constant  Value=[1.93744421913302655724464784725569188594818115234375;-0.378442660504472172533496632240712642669677734375;0.98525146912289696121689530627918429672718048095703125;0.1445840763452901633900893330064718611538410186767578125;0.7694976326429749935442714559030719101428985595703125;-1.6597322476003653068943322068662382662296295166015625;0.41488602467453594702107011471525765955448150634765625;-0.8708253961671073017924982195836491882801055908203125;0.59730623842644303689297657911083661019802093505859375;-0.7691421472733803721411049991729669272899627685546875;0.09497643588001160319667093290263437665998935699462890625;0.9641702161466974008163788312231190502643585205078125;0.106164476717207467704184864487615413963794708251953125;-0.66351410501644536577003918864647857844829559326171875;-0.156644952328087339044060399828595109283924102783203125]
      mask Display: e = 0.06;c1 = [120 150 230]/255;c2 = ([120 150 230]+0)/383;c3 = ([120 150 230]+128)/383;patch([0 1 1 0],[0 0 1 1],c1);patch([0 1 1 1-e 1-e 0+e],[0 0 1 1-e 0+e 0+e],c2);patch([0 0 1 1-e 0+e 0+e],[0 1 1 1-e 1-e 0+e],c3);plot([0 1 1 0 0],[0 0 1 1 0]);disp('weights');
  "IW{2,1}(22,:)'" : Constant  Value=[0.5453053215646843643327201789361424744129180908203125;-0.38125188591185599218391644171788357198238372802734375;-0.1442271338931526980520203551350277848541736602783203125;-0.341390807187336220440698753009201027452945709228515625;0.392205893042667452785821069483063183724880218505859375;-0.33758485444321795210242953544366173446178436279296875;-0.40462352785172683855563491306384094059467315673828125;-0.09289453296408155258401251330724335275590419769287109375;0.0178490816555314617264382803796252119354903697967529296875;0.376176695474876143787668070217478089034557342529296875;-0.67026136444375195022615798734477721154689788818359375;0.593903476576711053525059469393454492092132568359375;0.3497907813853746716858950094319880008697509765625;-0.684882265104075571571229374967515468597412109375;-0.7482522873427004395097128508496098220348358154296875]
      mask Display: e = 0.06;c1 = [120 150 230]/255;c2 = ([120 150 230]+0)/383;c3 = ([120 150 230]+128)/383;patch([0 1 1 0],[0 0 1 1],c1);patch([0 1 1 1-e 1-e 0+e],[0 0 1 1-e 0+e 0+e],c2);patch([0 0 1 1-e 0+e 0+e],[0 1 1 1-e 1-e 0+e],c3);plot([0 1 1 0 0],[0 0 1 1 0]);disp('weights');
  "IW{2,1}(23,:)'" : Constant  Value=[1.347974728751208939314665258280001580715179443359375;-0.0781294578443663123579199236701242625713348388671875;-0.568234552178519702891890119644813239574432373046875;-0.1879189483594107257236061059302301146090030670166015625;-0.67150732673056368060571230671484954655170440673828125;1.96643061009864172916650204570032656192779541015625;-1.43781271419940726019603971508331596851348876953125;-0.6574325654373092131521616465761326253414154052734375;-0.84052250648908233277012413964257575571537017822265625;0.58099880563414341150263453528168611228466033935546875;-0.318074890163388357411378137840074487030506134033203125;0.95804752232167633696491293449071235954761505126953125;-0.777877843451402650742920741322450339794158935546875;-0.51536629588794202749824080456164665520191192626953125;0.400403516582479690466556121464236639440059661865234375]
      mask Display: e = 0.06;c1 = [120 150 230]/255;c2 = ([120 150 230]+0)/383;c3 = ([120 150 230]+128)/383;patch([0 1 1 0],[0 0 1 1],c1);patch([0 1 1 1-e 1-e 0+e],[0 0 1 1-e 0+e 0+e],c2);patch([0 0 1 1-e 0+e 0+e],[0 1 1 1-e 1-e 0+e],c3);plot([0 1 1 0 0],[0 0 1 1 0]);disp('weights');
  "IW{2,1}(24,:)'" : Constant  Value=[0.0739331340712322815367230077754356898367404937744140625;-0.270922287657474336608487419653101824223995208740234375;-0.59803181901180824109331979343551211059093475341796875;0.8879290196003160051674285568878985941410064697265625;0.9267279593880910493197688992950133979320526123046875;-0.71741651912279735814337300325860269367694854736328125;-0.92051347463212407351562660551280714571475982666015625;0.310105545944360072585510579301626421511173248291015625;1.2610642922595911574745741745573468506336212158203125;0.426233494481498331740709772930131293833255767822265625;-0.2007684175223961864364952134565101005136966705322265625;-1.147196855864600184560231355135329067707061767578125;0.09451345367921970552771426810068078339099884033203125;0.82737459894130538362588822565157897770404815673828125;0.269841101548220774208886041378718800842761993408203125]
      mask Display: e = 0.06;c1 = [120 150 230]/255;c2 = ([120 150 230]+0)/383;c3 = ([120 150 230]+128)/383;patch([0 1 1 0],[0 0 1 1],c1);patch([0 1 1 1-e 1-e 0+e],[0 0 1 1-e 0+e 0+e],c2);patch([0 0 1 1-e 0+e 0+e],[0 1 1 1-e 1-e 0+e],c3);plot([0 1 1 0 0],[0 0 1 1 0]);disp('weights');
  "IW{2,1}(25,:)'" : Constant  Value=[-0.5767569229227074156796106763067655265331268310546875;2.202309810531996703275581239722669124603271484375;-1.83261520824125856421460412093438208103179931640625;-0.34420980923971711273878781867097131907939910888671875;0.78029983782180833973285416504950262606143951416015625;-1.77809759515669885132638228242285549640655517578125;-2.2123936189164137289253631024621427059173583984375;0.6818862110570520496111157626728527247905731201171875;1.2043771119164998761874585397890768945217132568359375;1.5882785261696914513862566309398971498012542724609375;-0.001914321151931910706955886070090855355374515056610107421875;0.348373984809347059243833655273192562162876129150390625;0.06173707660948167530445829243035404942929744720458984375;0.10563547337733698860962050503076170571148395538330078125;-0.192366971449558776807720050783245824277400970458984375]
      mask Display: e = 0.06;c1 = [120 150 230]/255;c2 = ([120 150 230]+0)/383;c3 = ([120 150 230]+128)/383;patch([0 1 1 0],[0 0 1 1],c1);patch([0 1 1 1-e 1-e 0+e],[0 0 1 1-e 0+e 0+e],c2);patch([0 0 1 1-e 0+e 0+e],[0 1 1 1-e 1-e 0+e],c3);plot([0 1 1 0 0],[0 0 1 1 0]);disp('weights');
  "IW{2,1}(3,:)'" : Constant  Value=[-2.86609244089906045616089613758958876132965087890625;0.5146491757761364471690512800705619156360626220703125;2.415267939649645700939117887173779308795928955078125;0.048016690401786972508535455972378258593380451202392578125;-1.231553110496797831530102484975941479206085205078125;3.2929317877227806121709363651461899280548095703125;2.1784685092413358376006726757623255252838134765625;-1.360975228856546426214890743722207844257354736328125;0.6250877925503741661117373951128683984279632568359375;0.486477237967935238760475158414919860661029815673828125;0.09710569948105869653165456156784784980118274688720703125;0.54438347000795561658748056288459338247776031494140625;-0.476726273958989976708977565067471005022525787353515625;-0.64575151769479599561663007989409379661083221435546875;-0.1575299823375164720573593513108789920806884765625]
      mask Display: e = 0.06;c1 = [120 150 230]/255;c2 = ([120 150 230]+0)/383;c3 = ([120 150 230]+128)/383;patch([0 1 1 0],[0 0 1 1],c1);patch([0 1 1 1-e 1-e 0+e],[0 0 1 1-e 0+e 0+e],c2);patch([0 0 1 1-e 0+e 0+e],[0 1 1 1-e 1-e 0+e],c3);plot([0 1 1 0 0],[0 0 1 1 0]);disp('weights');
  "IW{2,1}(4,:)'" : Constant  Value=[-0.75606119661078363680672964619589038193225860595703125;-0.1351983232907857102045312558402656577527523040771484375;1.1759385570005738141929896301007829606533050537109375;-1.9856897299026663450405294497613795101642608642578125;0.25127169994193609969812541748979128897190093994140625;-0.362837569010614535702785588000551797449588775634765625;0.11605780882943007858987272129525081254541873931884765625;-0.25506652670973795071773793097236193716526031494140625;-0.26761612296503434205163785009062848985195159912109375;-0.91173452849609348813686438006698153913021087646484375;0.521628851757685918499873878317885100841522216796875;0.16033928363443672449051291550858877599239349365234375;0.8794056664068887751994907375774346292018890380859375;0.65104672528363149996977199407410807907581329345703125;-0.305798350601000301640652878631954081356525421142578125]
      mask Display: e = 0.06;c1 = [120 150 230]/255;c2 = ([120 150 230]+0)/383;c3 = ([120 150 230]+128)/383;patch([0 1 1 0],[0 0 1 1],c1);patch([0 1 1 1-e 1-e 0+e],[0 0 1 1-e 0+e 0+e],c2);patch([0 0 1 1-e 0+e 0+e],[0 1 1 1-e 1-e 0+e],c3);plot([0 1 1 0 0],[0 0 1 1 0]);disp('weights');
  "IW{2,1}(5,:)'" : Constant  Value=[0.2084567277317424804916612401939346455037593841552734375;0.914830631056013476865018674288876354694366455078125;0.255554068077470886155566631714464165270328521728515625;-1.08965574204619297660201482358388602733612060546875;0.86862247157069949476948522715247236192226409912109375;-1.2528569085254857018441043692291714251041412353515625;-0.43875715848940310959136468227370642125606536865234375;0.25231376586373077675062859270838089287281036376953125;-0.9827411366423692840044168406166136264801025390625;-0.1330299394789041522724204469341202639043331146240234375;0.30501439581215539220693244715221226215362548828125;0.247500142536799028203375883094849996268749237060546875;-0.045402302991062924719667392992050736211240291595458984375;-0.72600167964628570249630001853802241384983062744140625;-0.67591987956941412818423486896790564060211181640625]
      mask Display: e = 0.06;c1 = [120 150 230]/255;c2 = ([120 150 230]+0)/383;c3 = ([120 150 230]+128)/383;patch([0 1 1 0],[0 0 1 1],c1);patch([0 1 1 1-e 1-e 0+e],[0 0 1 1-e 0+e 0+e],c2);patch([0 0 1 1-e 0+e 0+e],[0 1 1 1-e 1-e 0+e],c3);plot([0 1 1 0 0],[0 0 1 1 0]);disp('weights');
  "IW{2,1}(6,:)'" : Constant  Value=[0.258485732582182048400198937088134698569774627685546875;-1.5520561569960202863427412012242712080478668212890625;0.7561887717298734212789668163168244063854217529296875;-1.2208784831629337919167710424517281353473663330078125;0.697868240218944446695559236104600131511688232421875;0.31292175001746180829087506936048157513141632080078125;-0.3106340482992566709441462080576457083225250244140625;-0.425838574254970014809629219598718918859958648681640625;1.255036738243307414819582845666445791721343994140625;-0.5051407966406464833397649272228591144084930419921875;0.414314818602700529748261715212720446288585662841796875;0.82534871063334469543093518950627185404300689697265625;0.380530803229145841992675514120492152869701385498046875;0.15253976988195516728552547647268511354923248291015625;-0.7658982017002955444695544429123401641845703125]
      mask Display: e = 0.06;c1 = [120 150 230]/255;c2 = ([120 150 230]+0)/383;c3 = ([120 150 230]+128)/383;patch([0 1 1 0],[0 0 1 1],c1);patch([0 1 1 1-e 1-e 0+e],[0 0 1 1-e 0+e 0+e],c2);patch([0 0 1 1-e 0+e 0+e],[0 1 1 1-e 1-e 0+e],c3);plot([0 1 1 0 0],[0 0 1 1 0]);disp('weights');
  "IW{2,1}(7,:)'" : Constant  Value=[0.503321704807289993510721615166403353214263916015625;-0.39583682024811850386214473473955877125263214111328125;0.2963816754535419928373585207737050950527191162109375;-0.08870249654602598010644243231581640429794788360595703125;0.435265334634155343085382128265337087213993072509765625;-0.5999156399675167339324843851500190794467926025390625;0.5909163718124634812056683585979044437408447265625;-0.5664893524369214450331355692469514906406402587890625;-0.1547113923968227722216539632427156902849674224853515625;-0.52618096413273540701283081943984143435955047607421875;-0.62929024388621745966787557335919700562953948974609375;0.01140859063630311580339604660139229963533580303192138671875;-0.6643886397367595453289368379046209156513214111328125;0.57408129142878439044039851069101132452487945556640625;0.127987518088553187123324050844530574977397918701171875]
      mask Display: e = 0.06;c1 = [120 150 230]/255;c2 = ([120 150 230]+0)/383;c3 = ([120 150 230]+128)/383;patch([0 1 1 0],[0 0 1 1],c1);patch([0 1 1 1-e 1-e 0+e],[0 0 1 1-e 0+e 0+e],c2);patch([0 0 1 1-e 0+e 0+e],[0 1 1 1-e 1-e 0+e],c3);plot([0 1 1 0 0],[0 0 1 1 0]);disp('weights');
  "IW{2,1}(8,:)'" : Constant  Value=[-0.800274696627062187559431549743749201297760009765625;-1.1822721270319453967800882310257293283939361572265625;0.76134097237127973389902990675182081758975982666015625;-0.093663249778209001217277318573906086385250091552734375;0.017558301955229956015092085408468847163021564483642578125;-2.023311906094880985307327136979438364505767822265625;0.67424676535043914782363572157919406890869140625;0.955827515897161195113085341290570795536041259765625;-0.05173210987429410767646231761318631470203399658203125;0.4668956585477415099916242979816161096096038818359375;-0.30446860070097236938835294495220296084880828857421875;0.81109979504506901637483906597481109201908111572265625;0.3237143151131263163478024580399505794048309326171875;0.1800630629791604986333908300366601906716823577880859375;-0.362739812479735912464917646502726711332798004150390625]
      mask Display: e = 0.06;c1 = [120 150 230]/255;c2 = ([120 150 230]+0)/383;c3 = ([120 150 230]+128)/383;patch([0 1 1 0],[0 0 1 1],c1);patch([0 1 1 1-e 1-e 0+e],[0 0 1 1-e 0+e 0+e],c2);patch([0 0 1 1-e 0+e 0+e],[0 1 1 1-e 1-e 0+e],c3);plot([0 1 1 0 0],[0 0 1 1 0]);disp('weights');
  "IW{2,1}(9,:)'" : Constant  Value=[0.77694533171888380262970486000995151698589324951171875;-0.218725719907354398952037399794789962470531463623046875;-0.102783333869597204301982174001750536262989044189453125;-0.8826987866118944925375444654491730034351348876953125;-1.5483893437083022792677411416661925613880157470703125;0.94725386152138124629118465236388146877288818359375;-0.67773829325277679114236661916947923600673675537109375;-0.58984009689855276814540729901636950671672821044921875;1.1776973595169002440030681100324727594852447509765625;0.80273512282423775676676314105861820280551910400390625;0.64479838509049247630144918730366043746471405029296875;1.2963036605293629666135757361189462244510650634765625;-0.76173958941907382591551822770270518958568572998046875;-0.61927954450255573437544853732106275856494903564453125;-0.453152060244526477816862097824923694133758544921875]
      mask Display: e = 0.06;c1 = [120 150 230]/255;c2 = ([120 150 230]+0)/383;c3 = ([120 150 230]+128)/383;patch([0 1 1 0],[0 0 1 1],c1);patch([0 1 1 1-e 1-e 0+e],[0 0 1 1-e 0+e 0+e],c2);patch([0 0 1 1-e 0+e 0+e],[0 1 1 1-e 1-e 0+e],c3);plot([0 1 1 0 0],[0 0 1 1 0]);disp('weights');
  Mux : Mux  Inputs=25
      mask Display: e = 0.06;c1 = [120 150 230]/255;c2 = ([120 150 230]+0)/383;c3 = ([120 150 230]+128)/383;patch([0 1 1 0],[0 0 1 1],c1);patch([0 1 1 1-e 1-e 0+e],[0 0 1 1-e 0+e 0+e],c2);patch([0 0 1 1-e 0+e 0+e],[0 1 1 1-e 1-e 0+e],c3);plot([0 1 1 0 0],[0 0 1 1 0]);disp('Mux');
  dotprod{1..25} (25 alike) : neural/Weight Functions/dotprod
  "lz{2,1}" : Outport
      mask Display: e = 0.06;c1 = [120 230 180]/255;c2 = ([120 230 180]+0)/(256+128);c3 = ([120 230 180]+128)/(256+128);patch([0 1 1 0],[0 0 1 1],c1);patch([0 1 1 1-e 1-e 0+e],[0 0 1 1-e 0+e 0+e],c2);patch([0 0 1 1-e 0+e 0+e],[0 1 1 1-e 1-e 0+e],c3);plot([0 1 1 0 0],[0 0 1 1 0]);
  wires:
  "IW{2,1}(1,:)'"/1 -> dotprod1/1
  "ad{2,1}"/1 -> dotprod1/2, dotprod2/2, dotprod3/2, dotprod4/2, dotprod5/2, dotprod6/2, dotprod7/2, dotprod8/2, dotprod9/2, dotprod10/2, dotprod11/2, dotprod12/2, dotprod13/2, dotprod14/2, dotprod15/2, dotprod16/2, dotprod17/2, dotprod18/2, dotprod19/2, dotprod20/2, dotprod21/2, dotprod22/2, dotprod23/2, dotprod24/2, dotprod25/2
  dotprod1/1 -> Mux/1
  "IW{2,1}(2,:)'"/1 -> dotprod2/1
  dotprod2/1 -> Mux/2
  "IW{2,1}(3,:)'"/1 -> dotprod3/1
  dotprod3/1 -> Mux/3
  "IW{2,1}(4,:)'"/1 -> dotprod4/1
  dotprod4/1 -> Mux/4
  "IW{2,1}(5,:)'"/1 -> dotprod5/1
  dotprod5/1 -> Mux/5
  "IW{2,1}(6,:)'"/1 -> dotprod6/1
  dotprod6/1 -> Mux/6
  "IW{2,1}(7,:)'"/1 -> dotprod7/1
  dotprod7/1 -> Mux/7
  "IW{2,1}(8,:)'"/1 -> dotprod8/1
  dotprod8/1 -> Mux/8
  "IW{2,1}(9,:)'"/1 -> dotprod9/1
  dotprod9/1 -> Mux/9
  "IW{2,1}(10,:)'"/1 -> dotprod10/1
  dotprod10/1 -> Mux/10
  "IW{2,1}(11,:)'"/1 -> dotprod11/1
  dotprod11/1 -> Mux/11
  "IW{2,1}(12,:)'"/1 -> dotprod12/1
  dotprod12/1 -> Mux/12
  "IW{2,1}(13,:)'"/1 -> dotprod13/1
  dotprod13/1 -> Mux/13
  "IW{2,1}(14,:)'"/1 -> dotprod14/1
  dotprod14/1 -> Mux/14
  "IW{2,1}(15,:)'"/1 -> dotprod15/1
  dotprod15/1 -> Mux/15
  "IW{2,1}(16,:)'"/1 -> dotprod16/1
  dotprod16/1 -> Mux/16
  "IW{2,1}(17,:)'"/1 -> dotprod17/1
  dotprod17/1 -> Mux/17
  "IW{2,1}(18,:)'"/1 -> dotprod18/1
  dotprod18/1 -> Mux/18
  "IW{2,1}(19,:)'"/1 -> dotprod19/1
  dotprod19/1 -> Mux/19
  "IW{2,1}(20,:)'"/1 -> dotprod20/1
  dotprod20/1 -> Mux/20
  "IW{2,1}(21,:)'"/1 -> dotprod21/1
  dotprod21/1 -> Mux/21
  "IW{2,1}(22,:)'"/1 -> dotprod22/1
  dotprod22/1 -> Mux/22
  "IW{2,1}(23,:)'"/1 -> dotprod23/1
  dotprod23/1 -> Mux/23
  "IW{2,1}(24,:)'"/1 -> dotprod24/1
  dotprod24/1 -> Mux/24
  "IW{2,1}(25,:)'"/1 -> dotprod25/1
  dotprod25/1 -> Mux/25
  Mux/1 -> "lz{2,1}"/1

== system ackerman_ROS_neural_controller_v2/ME ENCANTA/Layer 3/Delays 1 ==
  "p{3}" : Inport  PortDimensions=25  SampleTime=0.1
      mask Display: e = 0.06;c1 = [120 230 180]/255;c2 = ([120 230 180]+0)/(256+128);c3 = ([120 230 180]+128)/(256+128);patch([0 1 1 0],[0 0 1 1],c1);patch([0 1 1 1-e 1-e 0+e],[0 0 1 1-e 0+e 0+e],c2);patch([0 0 1 1-e 0+e 0+e],[0 1 1 1-e 1-e 0+e],c3);plot([0 1 1 0 0],[0 0 1 1 0]);
  mux : Mux  Inputs=1
      mask Display: e = 0.06;c1 = [120 150 230]/255;c2 = ([120 150 230]+0)/383;c3 = ([120 150 230]+128)/383;patch([0 1 1 0],[0 0 1 1],c1);patch([0 1 1 1-e 1-e 0+e],[0 0 1 1-e 0+e 0+e],c2);patch([0 0 1 1-e 0+e 0+e],[0 1 1 1-e 1-e 0+e],c3);plot([0 1 1 0 0],[0 0 1 1 0]);disp('Mux')
  "pd{3,2}" : Outport
      mask Display: e = 0.06;c1 = [120 230 180]/255;c2 = ([120 230 180]+0)/(256+128);c3 = ([120 230 180]+128)/(256+128);patch([0 1 1 0],[0 0 1 1],c1);patch([0 1 1 1-e 1-e 0+e],[0 0 1 1-e 0+e 0+e],c2);patch([0 0 1 1-e 0+e 0+e],[0 1 1 1-e 1-e 0+e],c3);plot([0 1 1 0 0],[0 0 1 1 0]);
  wires:
  "p{3}"/1 -> mux/1
  mux/1 -> "pd{3,2}"/1
